simulink model "ev_cell_digital_twin"  (R2025b)
settings: Solver=ode45  StartTime=0.0  StopTime=10.0  MaxStep=0.005  RelTol=1e-3
settings Model: Creator=Santhosh  LastModifiedBy=Santhosh

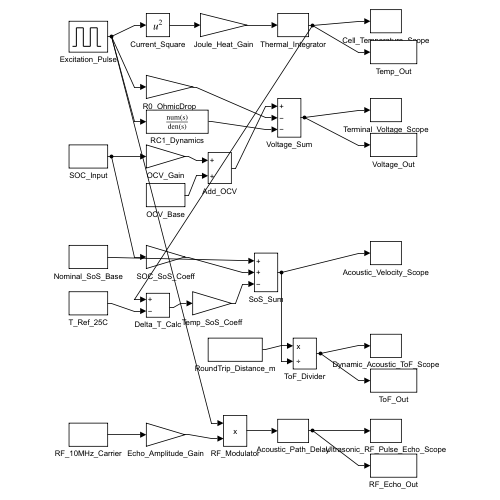
[thumbnail: Simulink's stored preview of the top-level diagram]
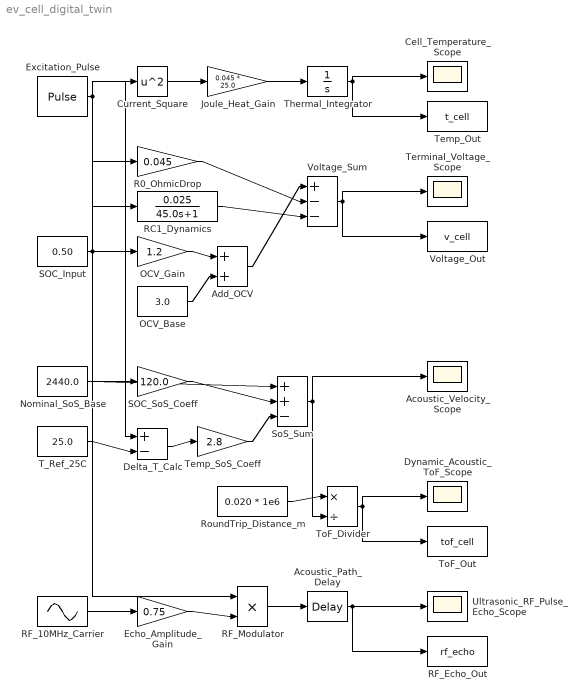
== system ev_cell_digital_twin ==
  Acoustic_Path_Delay : TransportDelay  DelayTime=0.008
  Acoustic_Velocity_Scope : Scope
  Add_OCV : Sum
  Cell_Temperature_Scope : Scope
  Current_Square : Math  Operator=square
  Delta_T_Calc : Sum  Inputs=+-
  Dynamic_Acoustic_ToF_Scope : Scope
  Echo_Amplitude_Gain : Gain  Gain=0.75
  Excitation_Pulse : DiscretePulseGenerator  PulseType=Time based  Amplitude=0.5  Period=1.0  PulseWidth=20
  Joule_Heat_Gain : Gain  Gain=0.045 * 25.0
  Nominal_SoS_Base : Constant  Value=2440.0
  OCV_Base : Constant  Value=3.0
  OCV_Gain : Gain  Gain=1.2
  R0_OhmicDrop : Gain  Gain=0.045
  RC1_Dynamics : TransferFcn  Numerator=[0.025]  Denominator=[45.0, 1]
  RF_10MHz_Carrier : Sin  Amplitude=1.0  Frequency=2*pi*5.0  SampleTime=0
  RF_Echo_Out : ToWorkspace  VariableName=rf_echo  SampleTime=-1
  RF_Modulator : Product  Inputs=**
  RoundTrip_Distance_m : Constant  Value=0.020 * 1e6
  SOC_Input : Constant  Value=0.50
  SOC_SoS_Coeff : Gain  Gain=120.0
  SoS_Sum : Sum  Inputs=++-
  T_Ref_25C : Constant  Value=25.0
  Temp_Out : ToWorkspace  VariableName=t_cell  SampleTime=-1
  Temp_SoS_Coeff : Gain  Gain=2.8
  Terminal_Voltage_Scope : Scope
  Thermal_Integrator : Integrator  InitialCondition=25.0
  ToF_Divider : Product  Inputs=*/
  ToF_Out : ToWorkspace  VariableName=tof_cell  SampleTime=-1
  Ultrasonic_RF_Pulse_Echo_Scope : Scope
  Voltage_Out : ToWorkspace  VariableName=v_cell  SampleTime=-1
  Voltage_Sum : Sum  Inputs=+--
  wires:
  Excitation_Pulse/1 -> Current_Square/1, R0_OhmicDrop/1, RC1_Dynamics/1, RF_Modulator/1
  Current_Square/1 -> Joule_Heat_Gain/1
  Joule_Heat_Gain/1 -> Thermal_Integrator/1
  Thermal_Integrator/1 -> Cell_Temperature_Scope/1, Temp_Out/1, Delta_T_Calc/1
  SOC_Input/1 -> OCV_Gain/1, SOC_SoS_Coeff/1
  OCV_Gain/1 -> Add_OCV/1
  OCV_Base/1 -> Add_OCV/2
  Add_OCV/1 -> Voltage_Sum/1
  R0_OhmicDrop/1 -> Voltage_Sum/2
  RC1_Dynamics/1 -> Voltage_Sum/3
  Voltage_Sum/1 -> Terminal_Voltage_Scope/1, Voltage_Out/1
  T_Ref_25C/1 -> Delta_T_Calc/2
  Delta_T_Calc/1 -> Temp_SoS_Coeff/1
  Nominal_SoS_Base/1 -> SoS_Sum/1
  SOC_SoS_Coeff/1 -> SoS_Sum/2
  Temp_SoS_Coeff/1 -> SoS_Sum/3
  SoS_Sum/1 -> Acoustic_Velocity_Scope/1, ToF_Divider/2
  RoundTrip_Distance_m/1 -> ToF_Divider/1
  ToF_Divider/1 -> Dynamic_Acoustic_ToF_Scope/1, ToF_Out/1
  RF_10MHz_Carrier/1 -> Echo_Amplitude_Gain/1
  Echo_Amplitude_Gain/1 -> RF_Modulator/2
  RF_Modulator/1 -> Acoustic_Path_Delay/1
  Acoustic_Path_Delay/1 -> Ultrasonic_RF_Pulse_Echo_Scope/1, RF_Echo_Out/1
